simulink model "MIMOController_statespace"  (R2015b)
settings: Solver=VariableStepAuto  StartTime=0.0  StopTime=Simulation_Time  RelTol=1e-3
values from neighbouring files (symbols this model uses):
  A = [0 1 0 0; 0 24.4 0 0; 0 0 0 1; 0 0 0 0]    [LinABCD.m]
  B = [0 0;12648.1 0; 0 0;-2011.69 -.444031]    [LinABCD.m]
  C = [1 0 0 0;0 0 1 0]    [LinABCD.m]
  K_bar1 = [K_bar(:,1:4)]    [LinABCD.m]
  K_bar2 = [-K_bar(:,5:6)]    [LinABCD.m]
  Simulation_step = 1    [LinABCD.m]
settings Model: Creator=dmartin_a  LastModifiedBy=dmartin_a

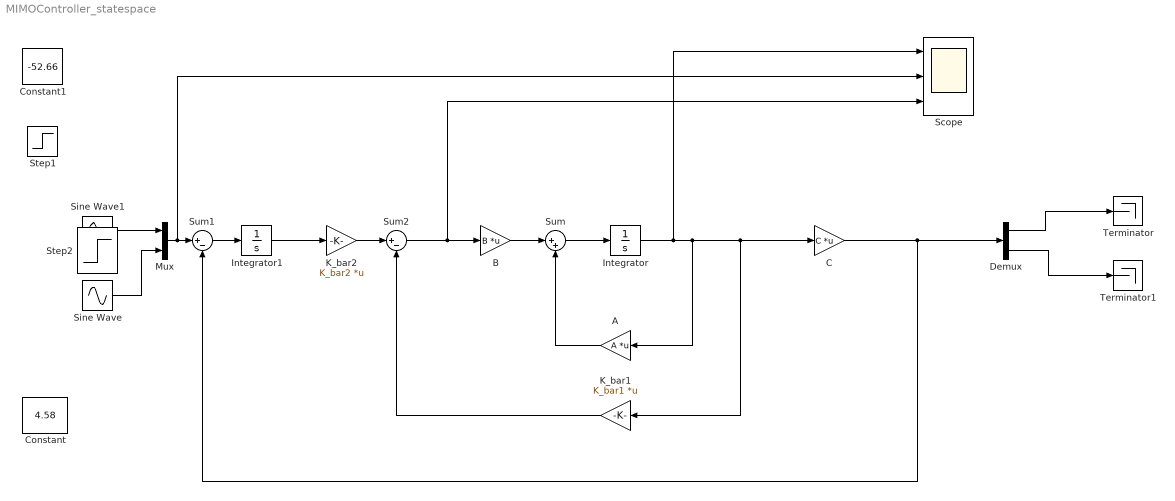
== system MIMOController_statespace ==
  A : Gain  Gain=A  Multiplication=Matrix(K*u)
  B : Gain  Gain=B  Multiplication=Matrix(K*u)
  C : Gain  Gain=C  Multiplication=Matrix(K*u)
  Constant : Constant  Value=4.58
  Constant1 : Constant  Value=-52.66
  Demux : Demux  Outputs=2
  Integrator : Integrator  InitialCondition=[0 0 0 0]
  Integrator1 : Integrator  InitialCondition=[0 0]
  K_bar1 : Gain  Gain=K_bar1  Multiplication=Matrix(K*u)
  K_bar2 : Gain  Gain=K_bar2  Multiplication=Matrix(K*u)
  Mux : Mux  Inputs=2
  Scope : Scope  NumInputPorts=3
  Sine Wave : Sin  SampleTime=0
  Sine Wave1 : Sin  SampleTime=0
  Step1 : Step  Time=100  Before=6  After=7  SampleTime=Simulation_step
  Step2 : Step  Time=100  Before=1  After=2  SampleTime=Simulation_step
  Sum : Sum  Inputs=|++
  Sum1 : Sum  Inputs=|+-
  Sum2 : Sum  Inputs=|+-
  Terminator : Terminator
  Terminator1 : Terminator
  wires:
  B/1 -> Sum/1
  Sum/1 -> Integrator/1
  Integrator/1 -> Scope/1, A/1, K_bar1/1, C/1
  A/1 -> Sum/2
  K_bar1/1 -> Sum2/2
  Sum2/1 -> Scope/3, B/1
  Demux/1 -> Terminator/1
  Demux/2 -> Terminator1/1
  C/1 -> Sum1/2, Demux/1
  Integrator1/1 -> K_bar2/1
  K_bar2/1 -> Sum2/1
  Mux/1 -> Scope/2, Sum1/1
  Sum1/1 -> Integrator1/1
  Sine Wave1/1 -> Mux/1
  Sine Wave/1 -> Mux/2
